simulink model "Motor_Pos_Simscape"  (R2014a)
settings: Solver=ode15s  StartTime=0.0  StopTime=5  RelTol=1e-3
values from neighbouring files (symbols this model uses):
  b = 3.5077e-6    (= 3.5077e-06)    [servo.m]
  J = 3.2284e-6    (= 3.2284e-06)    [servo.m]
  K = 0.0274    [servo.m]
  L = 2.75e-6    (= 2.75e-06)    [servo.m]
  R = 4    [servo.m]
libraries: simulink x1
settings Model: Creator=maen  LastModifiedBy=JinilGondalia
settings DataIOCC: SignalLoggingSaveFormat=ModelDataLogs
settings OptimizationCC: ExpressionDepthLimit=2147483647
settings DebuggingCC: UnderspecifiedInitializationDetection=Classic  FcnCallInpInsideContextMsg=UseLocalSettings  StateNameClashWarn=warning
settings GRTTargetCC: CombineOutputUpdateFcns=off  GRTInterface=on

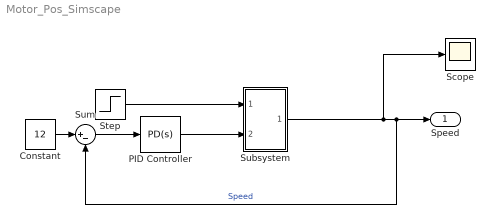
== system Motor_Pos_Simscape ==
  Constant : Constant  Value=12
  PID Controller : simulink/Continuous/PID Controller  Controller=PD  TimeDomain=Continuous-time  SampleTime=1  IntegratorMethod=Forward Euler  FilterMethod=Forward Euler  Form=Parallel  P=0.274108508408443  I=125.842386431999  D=0  N=100  InitialConditionSource=internal  InitialConditionForIntegrator=0  InitialConditionForFilter=0  ExternalReset=none  LimitOutput=off  UpperSaturationLimit=inf  LowerSaturationLimit=-inf  LinearizeAsGain=on  AntiWindupMode=none  Kb=1  TrackingMode=off  Kt=1  PParamMin=[]  PParamMax=[]  IParamMin=[]  IParamMax=[]  DParamMin=[]  DParamMax=[]  NParamMin=[]  NParamMax=[]  KbParamMin=[]  KbParamMax=[]  KtParamMin=[]  KtParamMax=[]  POutMin=[]  POutMax=[]  IOutMin=[]  IOutMax=[]  DOutMin=[]  DOutMax=[]  NOutMin=[]  NOutMax=[]  KbOutMin=[]  KbOutMax=[]  KtOutMin=[]  KtOutMax=[]  IntegratorOutMin=[]  IntegratorOutMax=[]  FilterOutMin=[]  FilterOutMax=[]  SumOutMin=[]  SumOutMax=[]  SumI1OutMin=[]  SumI1OutMax=[]  SumI2OutMin=[]  SumI2OutMax=[]  SumI3OutMin=[]  SumI3OutMax=[]  SumDOutMin=[]  SumDOutMax=[]  SaturationOutMin=[]  SaturationOutMax=[]  IntegratorContinuousStateAttributes=''  IntegratorStateMustResolveToSignalObject=off  IntegratorRTWStateStorageClass=Auto  FilterContinuousStateAttributes=''  FilterStateMustResolveToSignalObject=off  FilterRTWStateStorageClass=Auto
  Scope : Scope
      settings: SaveName=ScopeData3
  Step : Step  SampleTime=0
  Subsystem : Subsystem
  Sum : Sum  Inputs=|+-
  Speed : Outport
  wires:
  Subsystem/1(Speed1) -> Sum/2, Speed/1, Scope/1  "Speed"
  PID Controller/1 -> Subsystem/2(In2)
  Sum/1 -> PID Controller/1
  Constant/1 -> Sum/1
  Step/1 -> Subsystem/1(In1)

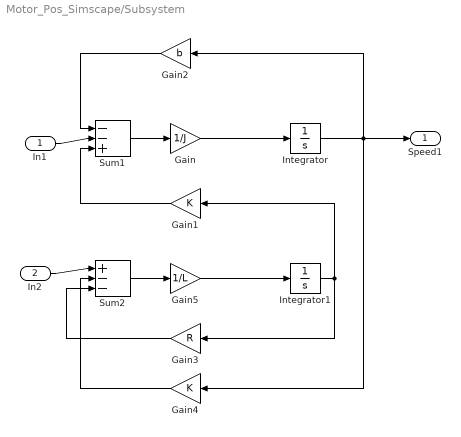
== system Motor_Pos_Simscape/Subsystem ==
  In1 : Inport
  In2 : Inport  Port=2
  Gain : Gain  Gain=1/J
  Gain1 : Gain  Gain=K
  Gain2 : Gain  Gain=b
  Gain3 : Gain  Gain=R
  Gain4 : Gain  Gain=K
  Gain5 : Gain  Gain=1/L
  Integrator : Integrator
  Integrator1 : Integrator
  Sum1 : Sum  Inputs=|--+
  Sum2 : Sum  Inputs=|+--
  Speed1 : Outport
  wires:
  Gain2/1 -> Sum1/1
  Gain3/1 -> Sum2/3
  Integrator1/1 -> Gain3/1, Gain1/1
  Sum2/1 -> Gain5/1
  Gain4/1 -> Sum2/2
  Gain1/1 -> Sum1/3
  Integrator/1 -> Speed1/1, Gain2/1, Gain4/1
  Sum1/1 -> Gain/1
  In1/1 -> Sum1/2
  Gain/1 -> Integrator/1
  Gain5/1 -> Integrator1/1
  In2/1 -> Sum2/1
